simulink model "robotarm_A2_pretrained"  (R2018b)
settings: Solver=FixedStepAuto  StartTime=0.0  StopTime=options.T_train  RelTol=1e-3  AbsTol=1e-6
undefined symbols (not defined in the file or in its folder): options
libraries: neural x132, simulink x2
(part 4 of 6)

== system robotarm_A2_pretrained/NN/Layer 3/Delays 1 ==
  "p{3}" : Inport  PortDimensions=30
      mask Display: e = 0.06;c1 = [120 230 180]/255;c2 = ([120 230 180]+0)/(256+128);c3 = ([120 230 180]+128)/(256+128);patch([0 1 1 0],[0 0 1 1],c1);patch([0 1 1 1-e 1-e 0+e],[0 0 1 1-e 0+e 0+e],c2);patch([0 0 1 1-e 0+e 0+e],[0 1 1 1-e 1-e 0+e],c3);plot([0 1 1 0 0],[0 0 1 1 0]);
  mux : Mux  Inputs=1
      mask Display: e = 0.06;c1 = [120 150 230]/255;c2 = ([120 150 230]+0)/383;c3 = ([120 150 230]+128)/383;patch([0 1 1 0],[0 0 1 1],c1);patch([0 1 1 1-e 1-e 0+e],[0 0 1 1-e 0+e 0+e],c2);patch([0 0 1 1-e 0+e 0+e],[0 1 1 1-e 1-e 0+e],c3);plot([0 1 1 0 0],[0 0 1 1 0]);disp('Mux')
  "pd{3,2}" : Outport
      mask Display: e = 0.06;c1 = [120 230 180]/255;c2 = ([120 230 180]+0)/(256+128);c3 = ([120 230 180]+128)/(256+128);patch([0 1 1 0],[0 0 1 1],c1);patch([0 1 1 1-e 1-e 0+e],[0 0 1 1-e 0+e 0+e],c2);patch([0 0 1 1-e 0+e 0+e],[0 1 1 1-e 1-e 0+e],c3);plot([0 1 1 0 0],[0 0 1 1 0]);
  wires:
  "p{3}"/1 -> mux/1
  mux/1 -> "pd{3,2}"/1

== system robotarm_A2_pretrained/NN/Layer 3/LW{3,2} ==
  "ad{3,2}" : Inport  PortDimensions=30
      mask Display: e = 0.06;c1 = [120 230 180]/255;c2 = ([120 230 180]+0)/(256+128);c3 = ([120 230 180]+128)/(256+128);patch([0 1 1 0],[0 0 1 1],c1);patch([0 1 1 1-e 1-e 0+e],[0 0 1 1-e 0+e 0+e],c2);patch([0 0 1 1-e 0+e 0+e],[0 1 1 1-e 1-e 0+e],c3);plot([0 1 1 0 0],[0 0 1 1 0]);
  "IW{3,2}(1,:)'" : Constant  Value=[-0.25694925165992865689901236692094244062900543212890625;0.1700539079035733591727108660052181221544742584228515625;-0.017125688246659144520211981443935655988752841949462890625;-0.315362693192650034301749428777839057147502899169921875;0.2154517218448439297429075622858363203704357147216796875;0.163819979801882953385216978858807124197483062744140625;0.39886275163531170750985666018095798790454864501953125;-0.398880943493153505841064543346874415874481201171875;0.255151735454595851582126897483249194920063018798828125;0.436896695589358952105385469621978700160980224609375;0.0080329063826333514664046475672876113094389438629150390625;-0.33026954113517426048218794676358811557292938232421875;-0.256286725335917342505354099557735025882720947265625;-0.60964324305010386684244849675451405346393585205078125;0.1429380799455385042673327689044526778161525726318359375;-0.269709600466735921475702753014047630131244659423828125;-0.034847005576559238193556922169591416604816913604736328125;-0.056374497690889154022375606700734351761639118194580078125;0.388106241384892081125457252710475586354732513427734375;-0.0722698510988753206607526635707472451031208038330078125;-0.3434244390093390553175822788034565746784210205078125;-0.18505252788413473208350978893577121198177337646484375;0.74635893658563812191886199798318557441234588623046875;-0.420940739625129956014149001930491067469120025634765625;0.33747178410502221002076339573250152170658111572265625;-0.491957705597507788386479887776658870279788970947265625;-0.07401590770908066108102474345287191681563854217529296875;-0.363093314476900019815985842797090299427509307861328125;-0.281917093729695145132296829615370370447635650634765625;0.01062811932019356621348382674341337406076490879058837890625]
      mask Display: e = 0.06;c1 = [120 150 230]/255;c2 = ([120 150 230]+0)/383;c3 = ([120 150 230]+128)/383;patch([0 1 1 0],[0 0 1 1],c1);patch([0 1 1 1-e 1-e 0+e],[0 0 1 1-e 0+e 0+e],c2);patch([0 0 1 1-e 0+e 0+e],[0 1 1 1-e 1-e 0+e],c3);plot([0 1 1 0 0],[0 0 1 1 0]);disp('weights');
  Mux : Mux  Inputs=1
      mask Display: e = 0.06;c1 = [120 150 230]/255;c2 = ([120 150 230]+0)/383;c3 = ([120 150 230]+128)/383;patch([0 1 1 0],[0 0 1 1],c1);patch([0 1 1 1-e 1-e 0+e],[0 0 1 1-e 0+e 0+e],c2);patch([0 0 1 1-e 0+e 0+e],[0 1 1 1-e 1-e 0+e],c3);plot([0 1 1 0 0],[0 0 1 1 0]);disp('Mux');
  dotprod1 : neural/Weight Functions/dotprod
  "lz{3,2}" : Outport
      mask Display: e = 0.06;c1 = [120 230 180]/255;c2 = ([120 230 180]+0)/(256+128);c3 = ([120 230 180]+128)/(256+128);patch([0 1 1 0],[0 0 1 1],c1);patch([0 1 1 1-e 1-e 0+e],[0 0 1 1-e 0+e 0+e],c2);patch([0 0 1 1-e 0+e 0+e],[0 1 1 1-e 1-e 0+e],c3);plot([0 1 1 0 0],[0 0 1 1 0]);
  wires:
  "IW{3,2}(1,:)'"/1 -> dotprod1/1
  "ad{3,2}"/1 -> dotprod1/2
  dotprod1/1 -> Mux/1
  Mux/1 -> "lz{3,2}"/1

== system robotarm_A2_pretrained/NN_cex_1/Layer 1/Delays 1 ==
  "p{1}" : Inport  PortDimensions=10
      mask Display: e = 0.06;c1 = [120 230 180]/255;c2 = ([120 230 180]+0)/(256+128);c3 = ([120 230 180]+128)/(256+128);patch([0 1 1 0],[0 0 1 1],c1);patch([0 1 1 1-e 1-e 0+e],[0 0 1 1-e 0+e 0+e],c2);patch([0 0 1 1-e 0+e 0+e],[0 1 1 1-e 1-e 0+e],c3);plot([0 1 1 0 0],[0 0 1 1 0]);
  mux : Mux  Inputs=1
      mask Display: e = 0.06;c1 = [120 150 230]/255;c2 = ([120 150 230]+0)/383;c3 = ([120 150 230]+128)/383;patch([0 1 1 0],[0 0 1 1],c1);patch([0 1 1 1-e 1-e 0+e],[0 0 1 1-e 0+e 0+e],c2);patch([0 0 1 1-e 0+e 0+e],[0 1 1 1-e 1-e 0+e],c3);plot([0 1 1 0 0],[0 0 1 1 0]);disp('Mux')
  "pd{1,1}" : Outport
      mask Display: e = 0.06;c1 = [120 230 180]/255;c2 = ([120 230 180]+0)/(256+128);c3 = ([120 230 180]+128)/(256+128);patch([0 1 1 0],[0 0 1 1],c1);patch([0 1 1 1-e 1-e 0+e],[0 0 1 1-e 0+e 0+e],c2);patch([0 0 1 1-e 0+e 0+e],[0 1 1 1-e 1-e 0+e],c3);plot([0 1 1 0 0],[0 0 1 1 0]);
  wires:
  "p{1}"/1 -> mux/1
  mux/1 -> "pd{1,1}"/1

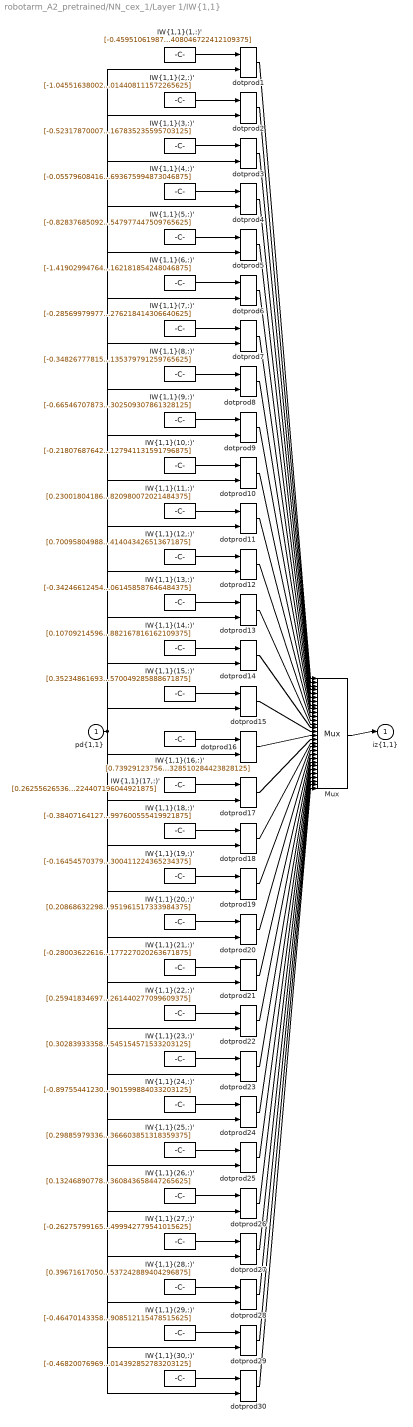
== system robotarm_A2_pretrained/NN_cex_1/Layer 1/IW{1,1} ==
  "pd{1,1}" : Inport  PortDimensions=10
      mask Display: e = 0.06;c1 = [120 230 180]/255;c2 = ([120 230 180]+0)/(256+128);c3 = ([120 230 180]+128)/(256+128);patch([0 1 1 0],[0 0 1 1],c1);patch([0 1 1 1-e 1-e 0+e],[0 0 1 1-e 0+e 0+e],c2);patch([0 0 1 1-e 0+e 0+e],[0 1 1 1-e 1-e 0+e],c3);plot([0 1 1 0 0],[0 0 1 1 0]);
  "IW{1,1}(1,:)'" : Constant  Value=[-0.4595106198764733473893784321262501180171966552734375;0.4454993566060585497012880296097137033939361572265625;-0.6086021933636562852854012817260809242725372314453125;0.09141764885368193482850784903348539955914020538330078125;-0.633250986270291083002348386798985302448272705078125;0.151795577324090213977569874259643256664276123046875;1.0426801816888602303379229851998388767242431640625;0.70670879616827153579805553818005137145519256591796875;1.124187654759598142817367261159233748912811279296875;0.45685376791020038123036783872521482408046722412109375]
      mask Display: e = 0.06;c1 = [120 150 230]/255;c2 = ([120 150 230]+0)/383;c3 = ([120 150 230]+128)/383;patch([0 1 1 0],[0 0 1 1],c1);patch([0 1 1 1-e 1-e 0+e],[0 0 1 1-e 0+e 0+e],c2);patch([0 0 1 1-e 0+e 0+e],[0 1 1 1-e 1-e 0+e],c3);plot([0 1 1 0 0],[0 0 1 1 0]);disp('Weights');
  "IW{1,1}(10,:)'" : Constant  Value=[-0.2180768764232653145196394461891031824052333831787109375;0.7809165792284680218671155671472661197185516357421875;0.39178217643791068969250090958666987717151641845703125;-0.73603218812764747980281754280440509319305419921875;0.338701286085252684099344833157374523580074310302734375;-0.408306761225813052984534579081810079514980316162109375;0.320152453482974996834542480428353883326053619384765625;0.9009715421136685886693840075167827308177947998046875;-0.4861484958899477959448631736449897289276123046875;-0.304716882155946944266133868950419127941131591796875]
      mask Display: e = 0.06;c1 = [120 150 230]/255;c2 = ([120 150 230]+0)/383;c3 = ([120 150 230]+128)/383;patch([0 1 1 0],[0 0 1 1],c1);patch([0 1 1 1-e 1-e 0+e],[0 0 1 1-e 0+e 0+e],c2);patch([0 0 1 1-e 0+e 0+e],[0 1 1 1-e 1-e 0+e],c3);plot([0 1 1 0 0],[0 0 1 1 0]);disp('Weights');
  "IW{1,1}(11,:)'" : Constant  Value=[0.23001804186197472024133503509801812469959259033203125;0.1638443570322423159524305447121150791645050048828125;-0.6530063781036250514233643116313032805919647216796875;0.141727193255944239336230339176836423575878143310546875;-0.52014353475075569832597466302104294300079345703125;0.425874550202590851366579727255157195031642913818359375;0.94190080379821117251282203142181970179080963134765625;-0.1985974577168597987597564724637777544558048248291015625;0.350760474937867439138017289224080741405487060546875;-0.5628610738455976925109780495404265820980072021484375]
      mask Display: e = 0.06;c1 = [120 150 230]/255;c2 = ([120 150 230]+0)/383;c3 = ([120 150 230]+128)/383;patch([0 1 1 0],[0 0 1 1],c1);patch([0 1 1 1-e 1-e 0+e],[0 0 1 1-e 0+e 0+e],c2);patch([0 0 1 1-e 0+e 0+e],[0 1 1 1-e 1-e 0+e],c3);plot([0 1 1 0 0],[0 0 1 1 0]);disp('Weights');
  "IW{1,1}(12,:)'" : Constant  Value=[0.7009580498866923026213271441520191729068756103515625;0.91400677494914506215906158104189671576023101806640625;-0.348781408993529440376590855521499179303646087646484375;-0.78662102315334314628358924892381764948368072509765625;-0.62865620584360371037035974950413219630718231201171875;-0.132248784270471653190526239995961077511310577392578125;0.064394466828491425669511727392091415822505950927734375;-0.503774620311830734209479487617500126361846923828125;-0.867044221350383725877009055693633854389190673828125;-0.30883663336519873165997296382556669414043426513671875]
      mask Display: e = 0.06;c1 = [120 150 230]/255;c2 = ([120 150 230]+0)/383;c3 = ([120 150 230]+128)/383;patch([0 1 1 0],[0 0 1 1],c1);patch([0 1 1 1-e 1-e 0+e],[0 0 1 1-e 0+e 0+e],c2);patch([0 0 1 1-e 0+e 0+e],[0 1 1 1-e 1-e 0+e],c3);plot([0 1 1 0 0],[0 0 1 1 0]);disp('Weights');
  "IW{1,1}(13,:)'" : Constant  Value=[-0.342466124542138261599433235460310243070125579833984375;0.553717638071313356107339131995104253292083740234375;-0.1133367538720705114396736234994023106992244720458984375;0.41927259693635132720146430074237287044525146484375;-0.86136786234662476857693036436103284358978271484375;1.028762466436916600542872402002103626728057861328125;0.81590966972469181062166398987756110727787017822265625;0.72099092004842468828229584687505848705768585205078125;0.448710055747644054324752005413756705820560455322265625;-0.435572645454710583035051740807830356061458587646484375]
      mask Display: e = 0.06;c1 = [120 150 230]/255;c2 = ([120 150 230]+0)/383;c3 = ([120 150 230]+128)/383;patch([0 1 1 0],[0 0 1 1],c1);patch([0 1 1 1-e 1-e 0+e],[0 0 1 1-e 0+e 0+e],c2);patch([0 0 1 1-e 0+e 0+e],[0 1 1 1-e 1-e 0+e],c3);plot([0 1 1 0 0],[0 0 1 1 0]);disp('Weights');
  "IW{1,1}(14,:)'" : Constant  Value=[0.107092145962798312996966387800057418644428253173828125;-0.76063293816721511131362376545439474284648895263671875;-0.5578939217263234606747346333577297627925872802734375;0.83695991117064794106994440880953334271907806396484375;-0.359335089622291992128566562314517796039581298828125;-0.5482026412963900696695418446324765682220458984375;0.550469020273391063113876953138969838619232177734375;0.1932055722064315583796911823810660280287265777587890625;0.057757038948209334094929801040052552707493305206298828125;-0.54135822735420580098519849343574605882167816162109375]
      mask Display: e = 0.06;c1 = [120 150 230]/255;c2 = ([120 150 230]+0)/383;c3 = ([120 150 230]+128)/383;patch([0 1 1 0],[0 0 1 1],c1);patch([0 1 1 1-e 1-e 0+e],[0 0 1 1-e 0+e 0+e],c2);patch([0 0 1 1-e 0+e 0+e],[0 1 1 1-e 1-e 0+e],c3);plot([0 1 1 0 0],[0 0 1 1 0]);disp('Weights');
  "IW{1,1}(15,:)'" : Constant  Value=[0.3523486169363481135263782562105916440486907958984375;0.63259405343298669155416291687288321554660797119140625;0.4078229877531873714957555421278811991214752197265625;-0.80651739097201324835140212599071674048900604248046875;-0.81861140573254231878053133186767809092998504638671875;0.37573878879080424564307350010494701564311981201171875;-0.63785872323546211060119048852357082068920135498046875;0.079261873363758172938986490407842211425304412841796875;-0.542934534749047070789629287901334464550018310546875;-0.4302861122866061815983584892819635570049285888671875]
      mask Display: e = 0.06;c1 = [120 150 230]/255;c2 = ([120 150 230]+0)/383;c3 = ([120 150 230]+128)/383;patch([0 1 1 0],[0 0 1 1],c1);patch([0 1 1 1-e 1-e 0+e],[0 0 1 1-e 0+e 0+e],c2);patch([0 0 1 1-e 0+e 0+e],[0 1 1 1-e 1-e 0+e],c3);plot([0 1 1 0 0],[0 0 1 1 0]);disp('Weights');
  "IW{1,1}(16,:)'" : Constant  Value=[0.7392912375678426517566776965395547449588775634765625;-0.439929644853198797971316480470704846084117889404296875;0.78532825618964607894412210953305475413799285888671875;-0.10515941990795507621214710525237023830413818359375;-1.0426793325453467264907203571056015789508819580078125;1.254082377134495107640077549149282276630401611328125;-0.69673410126086832150349437142722308635711669921875;0.30252367716362382754624604785931296646595001220703125;-0.1653322780654968848779162726714275777339935302734375;0.322476147973840554517011014468153007328510284423828125]
      mask Display: e = 0.06;c1 = [120 150 230]/255;c2 = ([120 150 230]+0)/383;c3 = ([120 150 230]+128)/383;patch([0 1 1 0],[0 0 1 1],c1);patch([0 1 1 1-e 1-e 0+e],[0 0 1 1-e 0+e 0+e],c2);patch([0 0 1 1-e 0+e 0+e],[0 1 1 1-e 1-e 0+e],c3);plot([0 1 1 0 0],[0 0 1 1 0]);disp('Weights');
  "IW{1,1}(17,:)'" : Constant  Value=[0.262556265364654872751515313211712054908275604248046875;0.401098003716192696987974386502173729240894317626953125;1.1604178344691382651632238776073791086673736572265625;-0.76362872981689855489406681954278610646724700927734375;0.1625780438632612179272740604574210010468959808349609375;-0.9786866435899652660879155519069172441959381103515625;-0.225197134339541804592954576946794986724853515625;0.6555612825211267757907762643299065530300140380859375;-0.52590308335115742988108422650839202105998992919921875;0.0437692115394376635162387856325949542224407196044921875]
      mask Display: e = 0.06;c1 = [120 150 230]/255;c2 = ([120 150 230]+0)/383;c3 = ([120 150 230]+128)/383;patch([0 1 1 0],[0 0 1 1],c1);patch([0 1 1 1-e 1-e 0+e],[0 0 1 1-e 0+e 0+e],c2);patch([0 0 1 1-e 0+e 0+e],[0 1 1 1-e 1-e 0+e],c3);plot([0 1 1 0 0],[0 0 1 1 0]);disp('Weights');
  "IW{1,1}(18,:)'" : Constant  Value=[-0.384071641276899022887647561219637282192707061767578125;1.01061087656192949424394100788049399852752685546875;-0.56400111704750643948358401758014224469661712646484375;0.039851310896567883335084303553230711258947849273681640625;0.210659065821322766254297675914131104946136474609375;-0.932956508738931322710641325102187693119049072265625;0.441795696991257924590712491408339701592922210693359375;0.05644222766016528114452199815787025727331638336181640625;-0.6115747681283958403497535982751287519931793212890625;-0.32686315219053063696463823362137190997600555419921875]
      mask Display: e = 0.06;c1 = [120 150 230]/255;c2 = ([120 150 230]+0)/383;c3 = ([120 150 230]+128)/383;patch([0 1 1 0],[0 0 1 1],c1);patch([0 1 1 1-e 1-e 0+e],[0 0 1 1-e 0+e 0+e],c2);patch([0 0 1 1-e 0+e 0+e],[0 1 1 1-e 1-e 0+e],c3);plot([0 1 1 0 0],[0 0 1 1 0]);disp('Weights');
  "IW{1,1}(19,:)'" : Constant  Value=[-0.164545703795691944382184601636254228651523590087890625;-0.06575842234431923671866826452969689853489398956298828125;-0.06493261374123766860311235404878971166908740997314453125;-0.903366752437792630558988093980588018894195556640625;0.0610753399756483739135859423186047933995723724365234375;-1.001372500557305755819470505230128765106201171875;0.0032440237331863041626844879061764004291035234928131103515625;0.63562309546348816358118938296684063971042633056640625;-0.8553097332503771799139258291688747704029083251953125;-0.79070121957604422302523516918881796300411224365234375]
      mask Display: e = 0.06;c1 = [120 150 230]/255;c2 = ([120 150 230]+0)/383;c3 = ([120 150 230]+128)/383;patch([0 1 1 0],[0 0 1 1],c1);patch([0 1 1 1-e 1-e 0+e],[0 0 1 1-e 0+e 0+e],c2);patch([0 0 1 1-e 0+e 0+e],[0 1 1 1-e 1-e 0+e],c3);plot([0 1 1 0 0],[0 0 1 1 0]);disp('Weights');
  "IW{1,1}(2,:)'" : Constant  Value=[-1.0455163800207103452777346319635398685932159423828125;1.1312154299509769028730943318805657327175140380859375;-0.7058290985517767790469179089996032416820526123046875;0.433560358991163352637698835678747855126857757568359375;-0.4151578323582858498497216714895330369472503662109375;-0.571800224434225956571253846050240099430084228515625;0.246478383218596608372763512306846678256988525390625;-0.10971565169970019792966553495716652832925319671630859375;0.169286786699414715240408213503542356193065643310546875;-1.3411075418972675521445125923492014408111572265625]
      mask Display: e = 0.06;c1 = [120 150 230]/255;c2 = ([120 150 230]+0)/383;c3 = ([120 150 230]+128)/383;patch([0 1 1 0],[0 0 1 1],c1);patch([0 1 1 1-e 1-e 0+e],[0 0 1 1-e 0+e 0+e],c2);patch([0 0 1 1-e 0+e 0+e],[0 1 1 1-e 1-e 0+e],c3);plot([0 1 1 0 0],[0 0 1 1 0]);disp('Weights');
  "IW{1,1}(20,:)'" : Constant  Value=[0.208686322981907979023930010953336022794246673583984375;0.01259019653386890015556165423049606033600866794586181640625;-0.68579631440263921771105515290400944650173187255859375;0.382506371563203384500440051851910538971424102783203125;0.64329879715530224881803178504924289882183074951171875;-0.05952835461690385299160510612637153826653957366943359375;0.42113479928850428013475948318955488502979278564453125;-0.4536767133101011761908694097655825316905975341796875;0.7940899476321547911794596075196750462055206298828125;-0.30221280394220373377578425788669846951961517333984375]
      mask Display: e = 0.06;c1 = [120 150 230]/255;c2 = ([120 150 230]+0)/383;c3 = ([120 150 230]+128)/383;patch([0 1 1 0],[0 0 1 1],c1);patch([0 1 1 1-e 1-e 0+e],[0 0 1 1-e 0+e 0+e],c2);patch([0 0 1 1-e 0+e 0+e],[0 1 1 1-e 1-e 0+e],c3);plot([0 1 1 0 0],[0 0 1 1 0]);disp('Weights');
  "IW{1,1}(21,:)'" : Constant  Value=[-0.280036226161772983100917144838604144752025604248046875;0.62556594768089646141362436537747271358966827392578125;0.1912613168033721333660679420063388533890247344970703125;-1.131163287794608063308032797067426145076751708984375;0.71941304697631947018265918813995085656642913818359375;1.0075993335810038420419232352287508547306060791015625;-0.1496041892429451347634739022396388463675975799560546875;0.79543461097307488483210136109846644103527069091796875;0.5065382525425388138273774529807269573211669921875;-0.1302350209670180003485029374132864177227020263671875]
      mask Display: e = 0.06;c1 = [120 150 230]/255;c2 = ([120 150 230]+0)/383;c3 = ([120 150 230]+128)/383;patch([0 1 1 0],[0 0 1 1],c1);patch([0 1 1 1-e 1-e 0+e],[0 0 1 1-e 0+e 0+e],c2);patch([0 0 1 1-e 0+e 0+e],[0 1 1 1-e 1-e 0+e],c3);plot([0 1 1 0 0],[0 0 1 1 0]);disp('Weights');
  "IW{1,1}(22,:)'" : Constant  Value=[0.259418346978302405414495979130151681602001190185546875;-0.0767351695005737688415337061087484471499919891357421875;-0.2380076007601285847936622985798749141395092010498046875;0.211239185297670051255636280984617769718170166015625;-0.86674739185102789296166747590177692472934722900390625;0.71416649781975405364420339537900872528553009033203125;0.465644308031372633482902756441035307943820953369140625;-0.545728417815332544904549649800173938274383544921875;-0.61414725227452160449814755338593386113643646240234375;0.638469082402826071387380579835735261440277099609375]
      mask Display: e = 0.06;c1 = [120 150 230]/255;c2 = ([120 150 230]+0)/383;c3 = ([120 150 230]+128)/383;patch([0 1 1 0],[0 0 1 1],c1);patch([0 1 1 1-e 1-e 0+e],[0 0 1 1-e 0+e 0+e],c2);patch([0 0 1 1-e 0+e 0+e],[0 1 1 1-e 1-e 0+e],c3);plot([0 1 1 0 0],[0 0 1 1 0]);disp('Weights');
  "IW{1,1}(23,:)'" : Constant  Value=[0.302839333583399927807278118052636273205280303955078125;-0.62352768411353720612311235527158714830875396728515625;-0.0589610859431066725022674290812574326992034912109375;0.28540701988521222087769046993344090878963470458984375;-0.64255265386347948375345140448189340531826019287109375;0.96491652552457229941040850462741218507289886474609375;0.2120810655044407522229477081054938025772571563720703125;-0.6727769805942924730146614820114336907863616943359375;0.182913231305678547489179663898539729416370391845703125;1.0990838958645252620982546432060189545154571533203125]
      mask Display: e = 0.06;c1 = [120 150 230]/255;c2 = ([120 150 230]+0)/383;c3 = ([120 150 230]+128)/383;patch([0 1 1 0],[0 0 1 1],c1);patch([0 1 1 1-e 1-e 0+e],[0 0 1 1-e 0+e 0+e],c2);patch([0 0 1 1-e 0+e 0+e],[0 1 1 1-e 1-e 0+e],c3);plot([0 1 1 0 0],[0 0 1 1 0]);disp('Weights');
  "IW{1,1}(24,:)'" : Constant  Value=[-0.8975544123049521427759600555873475968837738037109375;0.74493145571893448764200229561538435518741607666015625;-0.033874971310641655009021633304655551910400390625;-0.2912578974743642579170455064740963280200958251953125;-0.144967183870186977490135404877946712076663970947265625;0.65800847567882936317573694395832717418670654296875;-0.08481085689559052231967228863140917383134365081787109375;-0.8376253340980823747230488152126781642436981201171875;-0.41588743042776155078854571911506354808807373046875;-0.60492249224586924771784879339975304901599884033203125]
      mask Display: e = 0.06;c1 = [120 150 230]/255;c2 = ([120 150 230]+0)/383;c3 = ([120 150 230]+128)/383;patch([0 1 1 0],[0 0 1 1],c1);patch([0 1 1 1-e 1-e 0+e],[0 0 1 1-e 0+e 0+e],c2);patch([0 0 1 1-e 0+e 0+e],[0 1 1 1-e 1-e 0+e],c3);plot([0 1 1 0 0],[0 0 1 1 0]);disp('Weights');
  "IW{1,1}(25,:)'" : Constant  Value=[0.2988597933619718816089516622014343738555908203125;-0.90224952622846388283761598358978517353534698486328125;-0.55039751406182180204496035003103315830230712890625;-0.37110178113063529981019428305444307625293731689453125;0.80325492425276279195855977377505041658878326416015625;0.096388409289430432291823080959147773683071136474609375;-0.16219097083043620965980835535447113215923309326171875;0.475685969601705005427305650300695560872554779052734375;-0.71845298664056544968303796849795617163181304931640625;0.064175055566676630913747203521779738366603851318359375]
      mask Display: e = 0.06;c1 = [120 150 230]/255;c2 = ([120 150 230]+0)/383;c3 = ([120 150 230]+128)/383;patch([0 1 1 0],[0 0 1 1],c1);patch([0 1 1 1-e 1-e 0+e],[0 0 1 1-e 0+e 0+e],c2);patch([0 0 1 1-e 0+e 0+e],[0 1 1 1-e 1-e 0+e],c3);plot([0 1 1 0 0],[0 0 1 1 0]);disp('Weights');
  "IW{1,1}(26,:)'" : Constant  Value=[0.132468907785115830311184481615782715380191802978515625;-0.310943755922703457539313376400968991219997406005859375;-0.2907716634477235384537152640405111014842987060546875;-0.050869326242541805516150787980222958140075206756591796875;-0.79861410177234137819368697819299995899200439453125;0.4198376565088939305070425689336843788623809814453125;-0.79984383202196329687438947075861506164073944091796875;1.0692705330442837663440514006651937961578369140625;-0.8026144715751539759907018378726206719875335693359375;-0.34665774017511330473695352338836528360843658447265625]
      mask Display: e = 0.06;c1 = [120 150 230]/255;c2 = ([120 150 230]+0)/383;c3 = ([120 150 230]+128)/383;patch([0 1 1 0],[0 0 1 1],c1);patch([0 1 1 1-e 1-e 0+e],[0 0 1 1-e 0+e 0+e],c2);patch([0 0 1 1-e 0+e 0+e],[0 1 1 1-e 1-e 0+e],c3);plot([0 1 1 0 0],[0 0 1 1 0]);disp('Weights');
  "IW{1,1}(27,:)'" : Constant  Value=[-0.262757991650761579816020230282447300851345062255859375;0.35496239888055669542410441863466985523700714111328125;0.7464881210712304149268447872600518167018890380859375;0.455156181990929276093282851434196345508098602294921875;-0.278955522737699024293789307193947024643421173095703125;0.99274186956993359931544773644418455660343170166015625;0.88024020433884853087391775261494331061840057373046875;0.29923393557110566920442806804203428328037261962890625;-0.917410237536207429087653508759103715419769287109375;0.07606541966555424583162903218180872499942779541015625]
      mask Display: e = 0.06;c1 = [120 150 230]/255;c2 = ([120 150 230]+0)/383;c3 = ([120 150 230]+128)/383;patch([0 1 1 0],[0 0 1 1],c1);patch([0 1 1 1-e 1-e 0+e],[0 0 1 1-e 0+e 0+e],c2);patch([0 0 1 1-e 0+e 0+e],[0 1 1 1-e 1-e 0+e],c3);plot([0 1 1 0 0],[0 0 1 1 0]);disp('Weights');
  "IW{1,1}(28,:)'" : Constant  Value=[0.396716170501175857676656733019626699388027191162109375;-0.513702148120921631146984509541653096675872802734375;-0.64677070369960387719032723907730542123317718505859375;0.43260912281678221003033968372619710862636566162109375;-0.276790755307499802828630208750837482511997222900390625;-0.469675369772755424424559578255866654217243194580078125;0.1118674966534722869937468203715980052947998046875;0.92823775709025024838183526298962533473968505859375;-0.08142924889759262097044256734079681336879730224609375;0.8630196387956121650830709768342785537242889404296875]
      mask Display: e = 0.06;c1 = [120 150 230]/255;c2 = ([120 150 230]+0)/383;c3 = ([120 150 230]+128)/383;patch([0 1 1 0],[0 0 1 1],c1);patch([0 1 1 1-e 1-e 0+e],[0 0 1 1-e 0+e 0+e],c2);patch([0 0 1 1-e 0+e 0+e],[0 1 1 1-e 1-e 0+e],c3);plot([0 1 1 0 0],[0 0 1 1 0]);disp('Weights');
  "IW{1,1}(29,:)'" : Constant  Value=[-0.464701433585727630148909383933641947805881500244140625;-0.240499390494505582704931612170184962451457977294921875;-0.450335209921514822983823478352860547602176666259765625;0.986018401094572283227535081095993518829345703125;0.34314308179414643173998911152011714875698089599609375;0.5369216510935130859394348590285517275333404541015625;0.01047225811916151216873771545579074881970882415771484375;-0.1580015350896157022564381122720078565180301666259765625;0.9368616325747327611139780856319703161716461181640625;-0.6850782619353295022079919363022781908512115478515625]
      mask Display: e = 0.06;c1 = [120 150 230]/255;c2 = ([120 150 230]+0)/383;c3 = ([120 150 230]+128)/383;patch([0 1 1 0],[0 0 1 1],c1);patch([0 1 1 1-e 1-e 0+e],[0 0 1 1-e 0+e 0+e],c2);patch([0 0 1 1-e 0+e 0+e],[0 1 1 1-e 1-e 0+e],c3);plot([0 1 1 0 0],[0 0 1 1 0]);disp('Weights');
  "IW{1,1}(3,:)'" : Constant  Value=[-0.523178700077512104371635359711945056915283203125;0.82177392235693391686623954228707589209079742431640625;0.59209963227414241782042836348409764468669891357421875;0.485200440126057286338578933282406069338321685791015625;0.487399763124560791993644670583307743072509765625;0.5762417221555751201123030114104039967060089111328125;0.04247997481043992717975044115519267506897449493408203125;0.7330467916874017220152381923981010913848876953125;0.58906650250905101540155328621040098369121551513671875;0.51485391683193537648577375875902362167835235595703125]
      mask Display: e = 0.06;c1 = [120 150 230]/255;c2 = ([120 150 230]+0)/383;c3 = ([120 150 230]+128)/383;patch([0 1 1 0],[0 0 1 1],c1);patch([0 1 1 1-e 1-e 0+e],[0 0 1 1-e 0+e 0+e],c2);patch([0 0 1 1-e 0+e 0+e],[0 1 1 1-e 1-e 0+e],c3);plot([0 1 1 0 0],[0 0 1 1 0]);disp('Weights');
  "IW{1,1}(30,:)'" : Constant  Value=[-0.46820076969460477922524432869977317750453948974609375;0.55717128120582259942494829374481923878192901611328125;0.9290469391788824804478963415022008121013641357421875;0.470326127951398220705669928065617568790912628173828125;-0.275692773394275059128943894393160007894039154052734375;-0.2919807753210885703509802624466829001903533935546875;-0.62509172725765349554194472148083150386810302734375;-0.8614018173012072399075123030343092978000640869140625;-0.253655819037672147775452913265326060354709625244140625;0.038084651355074890244356566881833714433014392852783203125]
      mask Display: e = 0.06;c1 = [120 150 230]/255;c2 = ([120 150 230]+0)/383;c3 = ([120 150 230]+128)/383;patch([0 1 1 0],[0 0 1 1],c1);patch([0 1 1 1-e 1-e 0+e],[0 0 1 1-e 0+e 0+e],c2);patch([0 0 1 1-e 0+e 0+e],[0 1 1 1-e 1-e 0+e],c3);plot([0 1 1 0 0],[0 0 1 1 0]);disp('Weights');
  "IW{1,1}(4,:)'" : Constant  Value=[-0.055796084163377730746891103308371384628117084503173828125;0.70455884301178273165788823462207801640033721923828125;-0.11612120321176107318184023142748628742992877960205078125;0.75580131080242318741824192329659126698970794677734375;-0.59558685625206730929193099655094556510448455810546875;0.654175323953797072107363419490866363048553466796875;-0.1767496353810895926006452327783335931599140167236328125;-0.522628519375910816080477161449380218982696533203125;0.493459741356538528211927996380836702883243560791015625;-0.74632518487483689995087843271903693675994873046875]
      mask Display: e = 0.06;c1 = [120 150 230]/255;c2 = ([120 150 230]+0)/383;c3 = ([120 150 230]+128)/383;patch([0 1 1 0],[0 0 1 1],c1);patch([0 1 1 1-e 1-e 0+e],[0 0 1 1-e 0+e 0+e],c2);patch([0 0 1 1-e 0+e 0+e],[0 1 1 1-e 1-e 0+e],c3);plot([0 1 1 0 0],[0 0 1 1 0]);disp('Weights');
  "IW{1,1}(5,:)'" : Constant  Value=[-0.82837685092642232564941195960273034870624542236328125;0.1592759722046988846155812780125415883958339691162109375;-0.844622310567313405726963537745177745819091796875;0.917891266546870809861502493731677532196044921875;-0.30853021652315926193210771089070476591587066650390625;0.220530548606209519935106300181359983980655670166015625;-0.04254449685963125615817403968321741558611392974853515625;0.79948940237674293030067929066717624664306640625;-0.45542356238432757375989012871286831796169281005859375;0.266247470783954887085798191037611104547977447509765625]
      mask Display: e = 0.06;c1 = [120 150 230]/255;c2 = ([120 150 230]+0)/383;c3 = ([120 150 230]+128)/383;patch([0 1 1 0],[0 0 1 1],c1);patch([0 1 1 1-e 1-e 0+e],[0 0 1 1-e 0+e 0+e],c2);patch([0 0 1 1-e 0+e 0+e],[0 1 1 1-e 1-e 0+e],c3);plot([0 1 1 0 0],[0 0 1 1 0]);disp('Weights');
  "IW{1,1}(6,:)'" : Constant  Value=[-1.4190299476487613361541662015952169895172119140625;1.324273980566865294150602494482882320880889892578125;-0.2238178480457706231998571411168086342513561248779296875;0.2791849984976899623489998703007586300373077392578125;-0.799821971271625908883606825838796794414520263671875;0.8185142082673468877374034491367638111114501953125;0.29362093876172046247319258327479474246501922607421875;0.08344720819277150203330251088118529878556728363037109375;-0.0953290061726998760871509830394643358886241912841796875;0.60227907929938151454507533344440162181854248046875]
      mask Display: e = 0.06;c1 = [120 150 230]/255;c2 = ([120 150 230]+0)/383;c3 = ([120 150 230]+128)/383;patch([0 1 1 0],[0 0 1 1],c1);patch([0 1 1 1-e 1-e 0+e],[0 0 1 1-e 0+e 0+e],c2);patch([0 0 1 1-e 0+e 0+e],[0 1 1 1-e 1-e 0+e],c3);plot([0 1 1 0 0],[0 0 1 1 0]);disp('Weights');
  "IW{1,1}(7,:)'" : Constant  Value=[-0.285699799773916740530665947517263703048229217529296875;0.62359728120806756646032908975030295550823211669921875;0.29320290156767547795624295758898369967937469482421875;-0.343515406071193740711322561764973215758800506591796875;-0.42704081505023239184737349205533973872661590576171875;0.75111478494609984490892884423374198377132415771484375;0.61172288854854428574725488942931406199932098388671875;0.6812708431581828705247971811331808567047119140625;-0.1551824567007535626839143105826224200427532196044921875;-0.2164080541767467169567140672370442189276218414306640625]
      mask Display: e = 0.06;c1 = [120 150 230]/255;c2 = ([120 150 230]+0)/383;c3 = ([120 150 230]+128)/383;patch([0 1 1 0],[0 0 1 1],c1);patch([0 1 1 1-e 1-e 0+e],[0 0 1 1-e 0+e 0+e],c2);patch([0 0 1 1-e 0+e 0+e],[0 1 1 1-e 1-e 0+e],c3);plot([0 1 1 0 0],[0 0 1 1 0]);disp('Weights');
  "IW{1,1}(8,:)'" : Constant  Value=[-0.348267778153218465764240363569115288555622100830078125;-0.37812589344314095907151340725249610841274261474609375;-0.2823386412723587479689513202174566686153411865234375;0.56694318662727527513567338246502913534641265869140625;0.67425286949227736243983599706552922725677490234375;0.84470139110727426867697431589476764202117919921875;-0.6228211162190986360798206078470684587955474853515625;-0.6526596430086903932732411703909747302532196044921875;0.1921254072335736307053366545005701482295989990234375;-0.6868611876964385576371796560124494135379791259765625]
      mask Display: e = 0.06;c1 = [120 150 230]/255;c2 = ([120 150 230]+0)/383;c3 = ([120 150 230]+128)/383;patch([0 1 1 0],[0 0 1 1],c1);patch([0 1 1 1-e 1-e 0+e],[0 0 1 1-e 0+e 0+e],c2);patch([0 0 1 1-e 0+e 0+e],[0 1 1 1-e 1-e 0+e],c3);plot([0 1 1 0 0],[0 0 1 1 0]);disp('Weights');
  "IW{1,1}(9,:)'" : Constant  Value=[-0.66546707873781218989250874074059538543224334716796875;0.6008846289022093944964808542863465845584869384765625;-0.2906338810604740530152412247844040393829345703125;0.3217968203023595652467747640912421047687530517578125;-0.047339359250557218328214759139882517047226428985595703125;-0.75503388910941160450107645374373532831668853759765625;0.85958723103823919675647857729927636682987213134765625;-0.476412065556756914030955840644310228526592254638671875;0.1792174657227025846850665402598679065704345703125;-0.70907270763818275316481276604463346302509307861328125]
      mask Display: e = 0.06;c1 = [120 150 230]/255;c2 = ([120 150 230]+0)/383;c3 = ([120 150 230]+128)/383;patch([0 1 1 0],[0 0 1 1],c1);patch([0 1 1 1-e 1-e 0+e],[0 0 1 1-e 0+e 0+e],c2);patch([0 0 1 1-e 0+e 0+e],[0 1 1 1-e 1-e 0+e],c3);plot([0 1 1 0 0],[0 0 1 1 0]);disp('Weights');
  Mux : Mux  Inputs=30
      mask Display: e = 0.06;c1 = [120 150 230]/255;c2 = ([120 150 230]+0)/383;c3 = ([120 150 230]+128)/383;patch([0 1 1 0],[0 0 1 1],c1);patch([0 1 1 1-e 1-e 0+e],[0 0 1 1-e 0+e 0+e],c2);patch([0 0 1 1-e 0+e 0+e],[0 1 1 1-e 1-e 0+e],c3);plot([0 1 1 0 0],[0 0 1 1 0]);disp('Mux');
  dotprod{1..30} (30 alike) : neural/Weight Functions/dotprod
  "iz{1,1}" : Outport
      mask Display: e = 0.06;c1 = [120 230 180]/255;c2 = ([120 230 180]+0)/(256+128);c3 = ([120 230 180]+128)/(256+128);patch([0 1 1 0],[0 0 1 1],c1);patch([0 1 1 1-e 1-e 0+e],[0 0 1 1-e 0+e 0+e],c2);patch([0 0 1 1-e 0+e 0+e],[0 1 1 1-e 1-e 0+e],c3);plot([0 1 1 0 0],[0 0 1 1 0]);
  wires:
  "IW{1,1}(1,:)'"/1 -> dotprod1/1
  "pd{1,1}"/1 -> dotprod1/2, dotprod2/2, dotprod3/2, dotprod4/2, dotprod5/2, dotprod6/2, dotprod7/2, dotprod8/2, dotprod9/2, dotprod10/2, dotprod11/2, dotprod12/2, dotprod13/2, dotprod14/2, dotprod15/2, dotprod16/2, dotprod17/2, dotprod18/2, dotprod19/2, dotprod20/2, dotprod21/2, dotprod22/2, dotprod23/2, dotprod24/2, dotprod25/2, dotprod26/2, dotprod27/2, dotprod28/2, dotprod29/2, dotprod30/2
  dotprod1/1 -> Mux/1
  "IW{1,1}(2,:)'"/1 -> dotprod2/1
  dotprod2/1 -> Mux/2
  "IW{1,1}(3,:)'"/1 -> dotprod3/1
  dotprod3/1 -> Mux/3
  "IW{1,1}(4,:)'"/1 -> dotprod4/1
  dotprod4/1 -> Mux/4
  "IW{1,1}(5,:)'"/1 -> dotprod5/1
  dotprod5/1 -> Mux/5
  "IW{1,1}(6,:)'"/1 -> dotprod6/1
  dotprod6/1 -> Mux/6
  "IW{1,1}(7,:)'"/1 -> dotprod7/1
  dotprod7/1 -> Mux/7
  "IW{1,1}(8,:)'"/1 -> dotprod8/1
  dotprod8/1 -> Mux/8
  "IW{1,1}(9,:)'"/1 -> dotprod9/1
  dotprod9/1 -> Mux/9
  "IW{1,1}(10,:)'"/1 -> dotprod10/1
  dotprod10/1 -> Mux/10
  "IW{1,1}(11,:)'"/1 -> dotprod11/1
  dotprod11/1 -> Mux/11
  "IW{1,1}(12,:)'"/1 -> dotprod12/1
  dotprod12/1 -> Mux/12
  "IW{1,1}(13,:)'"/1 -> dotprod13/1
  dotprod13/1 -> Mux/13
  "IW{1,1}(14,:)'"/1 -> dotprod14/1
  dotprod14/1 -> Mux/14
  "IW{1,1}(15,:)'"/1 -> dotprod15/1
  dotprod15/1 -> Mux/15
  "IW{1,1}(16,:)'"/1 -> dotprod16/1
  dotprod16/1 -> Mux/16
  "IW{1,1}(17,:)'"/1 -> dotprod17/1
  dotprod17/1 -> Mux/17
  "IW{1,1}(18,:)'"/1 -> dotprod18/1
  dotprod18/1 -> Mux/18
  "IW{1,1}(19,:)'"/1 -> dotprod19/1
  dotprod19/1 -> Mux/19
  "IW{1,1}(20,:)'"/1 -> dotprod20/1
  dotprod20/1 -> Mux/20
  "IW{1,1}(21,:)'"/1 -> dotprod21/1
  dotprod21/1 -> Mux/21
  "IW{1,1}(22,:)'"/1 -> dotprod22/1
  dotprod22/1 -> Mux/22
  "IW{1,1}(23,:)'"/1 -> dotprod23/1
  dotprod23/1 -> Mux/23
  "IW{1,1}(24,:)'"/1 -> dotprod24/1
  dotprod24/1 -> Mux/24
  "IW{1,1}(25,:)'"/1 -> dotprod25/1
  dotprod25/1 -> Mux/25
  "IW{1,1}(26,:)'"/1 -> dotprod26/1
  dotprod26/1 -> Mux/26
  "IW{1,1}(27,:)'"/1 -> dotprod27/1
  dotprod27/1 -> Mux/27
  "IW{1,1}(28,:)'"/1 -> dotprod28/1
  dotprod28/1 -> Mux/28
  "IW{1,1}(29,:)'"/1 -> dotprod29/1
  dotprod29/1 -> Mux/29
  "IW{1,1}(30,:)'"/1 -> dotprod30/1
  dotprod30/1 -> Mux/30
  Mux/1 -> "iz{1,1}"/1

== system robotarm_A2_pretrained/NN_cex_1/Layer 2/Delays 1 ==
  "p{2}" : Inport  PortDimensions=30
      mask Display: e = 0.06;c1 = [120 230 180]/255;c2 = ([120 230 180]+0)/(256+128);c3 = ([120 230 180]+128)/(256+128);patch([0 1 1 0],[0 0 1 1],c1);patch([0 1 1 1-e 1-e 0+e],[0 0 1 1-e 0+e 0+e],c2);patch([0 0 1 1-e 0+e 0+e],[0 1 1 1-e 1-e 0+e],c3);plot([0 1 1 0 0],[0 0 1 1 0]);
  mux : Mux  Inputs=1
      mask Display: e = 0.06;c1 = [120 150 230]/255;c2 = ([120 150 230]+0)/383;c3 = ([120 150 230]+128)/383;patch([0 1 1 0],[0 0 1 1],c1);patch([0 1 1 1-e 1-e 0+e],[0 0 1 1-e 0+e 0+e],c2);patch([0 0 1 1-e 0+e 0+e],[0 1 1 1-e 1-e 0+e],c3);plot([0 1 1 0 0],[0 0 1 1 0]);disp('Mux')
  "pd{2,1}" : Outport
      mask Display: e = 0.06;c1 = [120 230 180]/255;c2 = ([120 230 180]+0)/(256+128);c3 = ([120 230 180]+128)/(256+128);patch([0 1 1 0],[0 0 1 1],c1);patch([0 1 1 1-e 1-e 0+e],[0 0 1 1-e 0+e 0+e],c2);patch([0 0 1 1-e 0+e 0+e],[0 1 1 1-e 1-e 0+e],c3);plot([0 1 1 0 0],[0 0 1 1 0]);
  wires:
  "p{2}"/1 -> mux/1
  mux/1 -> "pd{2,1}"/1
